simulink model "raman"  (R2024b)
settings: Solver=VariableStepAuto  StartTime=0.0  StopTime=20  RelTol=1e-3
values from neighbouring files (symbols this model uses):
  P0_laser = 70e-3    (= 0.07)    [Inverter_new.m]    (also in init_pv_inverter.m = 0.1)
  PRF = 10e3    (= 10000)    [Inverter_new.m]    (also in init_pv_inverter.m)
  RTI = 90    [init_pv_inverter.m]
  tau_p = 2*n_g*dz_DTS/c0    [Inverter_new.m]    (also in init_pv_inverter.m = 5e-09)
settings Model: Creator=tf  LastModifiedBy=tf

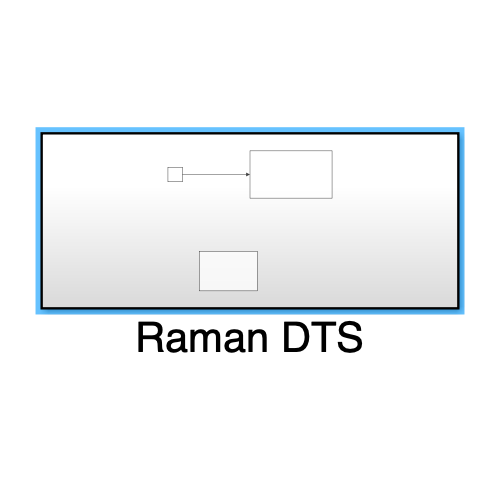
[thumbnail: Simulink's stored preview of the top-level diagram]
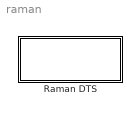
== system raman ==
  Raman DTS : Subsystem

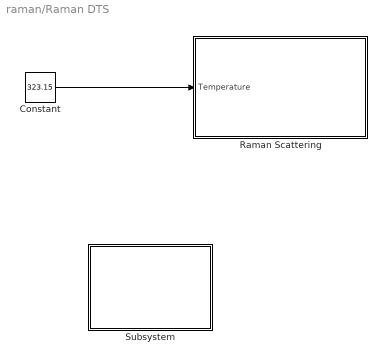
== system raman/Raman DTS ==
  Constant : Constant  Value=323.15
  Raman Scattering : Subsystem
  Subsystem : Subsystem
  wires:
  Constant/1 -> Raman Scattering/1(Temperature)

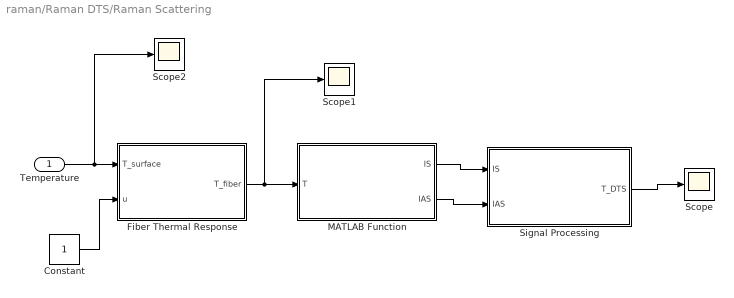
== system raman/Raman DTS/Raman Scattering ==
  Temperature : Inport
  Constant : Constant
  Fiber Thermal Response : Subsystem
  MATLAB Function : MATLAB Function  TreatAsAtomicUnit=on
  Scope : Scope
  Scope1 : Scope
  Scope2 : Scope
  Signal Processing : Subsystem
  wires:
  MATLAB Function/1(IS) -> Signal Processing/1(IS)
  MATLAB Function/2(IAS) -> Signal Processing/2(IAS)
  Signal Processing/1(T_DTS) -> Scope/1
  Constant/1 -> Fiber Thermal Response/2(u)
  Fiber Thermal Response/1(T_fiber) -> Scope1/1, MATLAB Function/1(T)
  Temperature/1 -> Scope2/1, Fiber Thermal Response/1(T_surface)

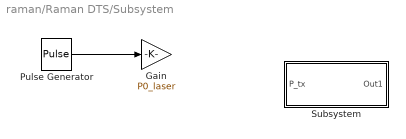
== system raman/Raman DTS/Subsystem ==
  Gain : Gain  Gain=P0_laser
  Pulse Generator : DiscretePulseGenerator  PulseType=Time based  Period=1/PRF  PulseWidth=100*tau_p*PRF
  Subsystem : Subsystem
  wires:
  Pulse Generator/1 -> Gain/1

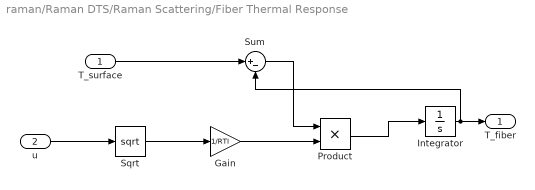
== system raman/Raman DTS/Raman Scattering/Fiber Thermal Response ==
  T_surface : Inport
  u : Inport  Port=2
  Gain : Gain  Gain=1/RTI
  Integrator : Integrator  InitialCondition=298.15
  Product : Product
  Sqrt : Sqrt
  Sum : Sum  Inputs=|+-
  T_fiber : Outport
  wires:
  u/1 -> Sqrt/1
  Gain/1 -> Product/2
  Sqrt/1 -> Gain/1
  T_surface/1 -> Sum/1
  Integrator/1 -> Sum/2, T_fiber/1
  Sum/1 -> Product/1
  Product/1 -> Integrator/1

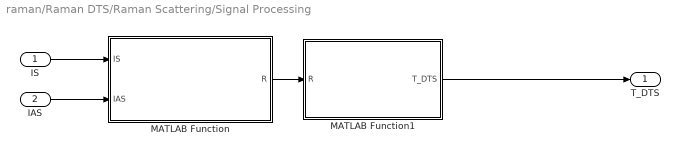
== system raman/Raman DTS/Raman Scattering/Signal Processing ==
  IS : Inport
  IAS : Inport  Port=2
  MATLAB Function : MATLAB Function  TreatAsAtomicUnit=on
  MATLAB Function1 : MATLAB Function  TreatAsAtomicUnit=on
  T_DTS : Outport
  wires:
  IS/1 -> MATLAB Function/1(IS)
  IAS/1 -> MATLAB Function/2(IAS)
  MATLAB Function/1(R) -> MATLAB Function1/1(R)
  MATLAB Function1/1(T_DTS) -> T_DTS/1

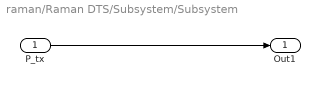
== system raman/Raman DTS/Subsystem/Subsystem ==
  P_tx : Inport
  Out1 : Outport
  wires:
  P_tx/1 -> Out1/1

== matlab function raman/Raman DTS/Raman Scattering/MATLAB Function ==
  data: T input; IS output; IAS output

function [IS, IAS] = RamanScattering(T)
%#codegen

IS = 0;
IAS = 0;

%Bose Einstein Phonon Occupancy Equation

h = 6.62607015 * 10^-34; % Plancks Constant
c = 299792458; % Speed of light
kB = 1.380649 * 10^-23; % Boltzmann Constant

%Raman Shift for Silica Based Materials

raman_shift_cm = 440; % Check this value
raman_shift_m = raman_shift_cm * 100;

%Raman Characteristics Temperature
thetaR = h*c*raman_shift_m/kB;

% Prevent invalid temperature values
T_safe = max(T, 1.0);

%Einstein Bose Equation

nPh = 1/(exp(thetaR/T_safe)-1);


% Raman intensities

IS  = nPh + 1;
IAS = nPh;

== matlab function raman/Raman DTS/Raman Scattering/Signal Processing/MATLAB Function1 ==
  data: R input; T_DTS output
function T_DTS = Reconstruct_Temperature(R)

%#codegen

%constants
h = 6.62607015 * 10^-34; % Plancks Constant
c = 299792458; % Speed of light
kB = 1.380649 * 10^-23; % Boltzmann Constant

% Raman shift for silica
raman_shift_cm = 440;                   % [cm^-1]
raman_shift_m  = raman_shift_cm * 100;  % [m^-1]

% Prevent invalid logarithm values
R_safe = min(max(R, 1e-12), 1 - 1e-12);

% Temperature reconstruction
T_DTS = -(h*c*raman_shift_m) / (kB*log(R_safe));

end

== matlab function raman/Raman DTS/Raman Scattering/Signal Processing/MATLAB Function ==
  data: IS input; R output; IAS input
function R = RamanRatio(IS, IAS)
%#codegen


%Safeguard to prevent division by zero
IS = max(IS,1e-12);


R = IAS/IS;

end
